simulink model "MultidifusionMensajes"  (R2023b)
settings: Solver=VariableStepAuto  StartTime=0.0  StopTime=10.0  RelTol=1e-3
settings Model: Creator=alfre  LastModifiedBy=alfre

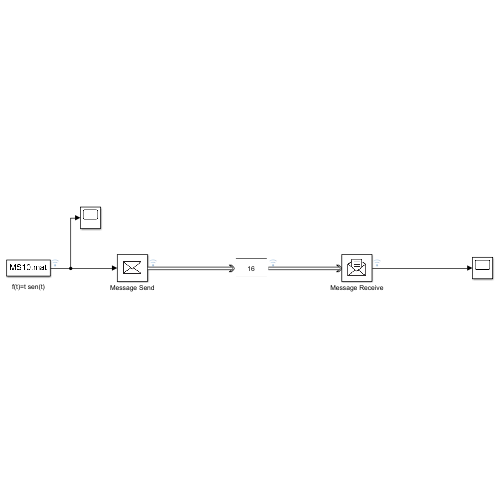
[thumbnail: Simulink's stored preview of the top-level diagram]
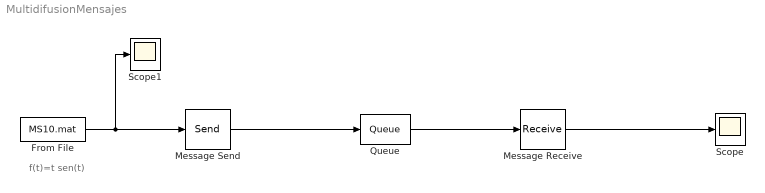
== system MultidifusionMensajes ==
  note: f(t)=t sen(t)
  From File : FromFile  FileName=MS10.mat  SampleTime=0
  Message Receive : Receive  InputPortMessageModes=m  SampleTime=0.1
  Message Send : Send  OutputPortMessageModes=m
  Queue : Queue  InputPortMessageModes=m  OutputPortMessageModes=m  OverwriteOldest=on  Capacity=16
  Scope : Scope
  Scope1 : Scope
  wires:
  From File/1 -> Scope1/1, Message Send/1
  Message Send/1 -> Queue/1
  Queue/1 -> Message Receive/1
  Message Receive/1 -> Scope/1
